simulink model "getTorque"  (R2021a)
settings: Solver=VariableStepAuto  StartTime=0.0  StopTime=10.0  RelTol=1e-3
libraries: cstblocks x1
settings Model: Creator=zande  LastModifiedBy=zande

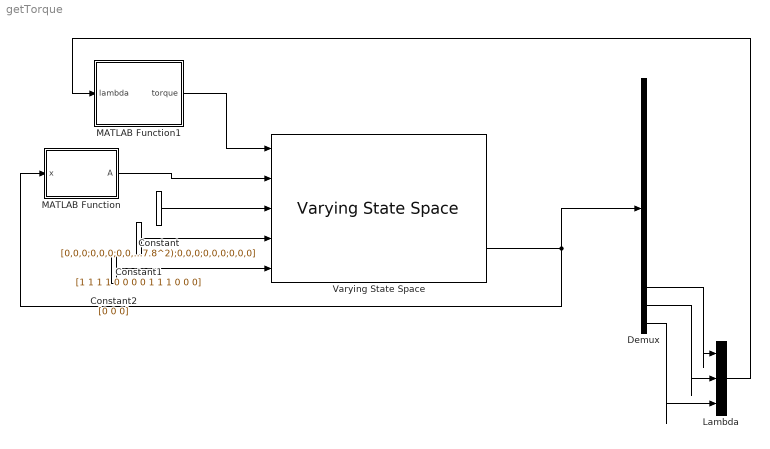
== system getTorque ==
  Constant : Constant  Value=[0,0,0;0,0,0;0,0,0;0,0,0;0,0,0;0,0,0;0,0,0;0,0,0;1/(396.2^2),0,0;0,1/(1867^2),0;0,0,1/(1987.8^2);0,0,0;0,0,0;0,0,0]
  Constant1 : Constant  Value=[1 1 1 1 0 0 0 0 1 1 1 0 0 0]
  Constant2 : Constant  Value=[0 0 0]
  Demux : Demux  Outputs=14
  Lambda : Mux  Inputs=3
  MATLAB Function : MATLAB Function  TreatAsAtomicUnit=on
  MATLAB Function1 : MATLAB Function  TreatAsAtomicUnit=on
  Varying State Space : cstblocks/Linear Parameter Varying/Varying State Space  x0=[2;2;2;2;2;2;.25;.25;.25;.25;.25;.25;2;2]  xNames=''  OutputX=on  OutputDX=off
  wires:
  MATLAB Function/1(A) -> Varying State Space/2
  Varying State Space/2 -> Demux/1, MATLAB Function/1(x)
  Demux/14 -> Lambda/3
  Lambda/1 -> MATLAB Function1/1(lambda)
  MATLAB Function1/1(torque) -> Varying State Space/1
  Constant/1 -> Varying State Space/3
  Constant1/1 -> Varying State Space/4
  Constant2/1 -> Varying State Space/5
  Demux/13 -> Lambda/2
  Demux/12 -> Lambda/1

== matlab function getTorque/MATLAB Function ==
  data: x input size=14;1; A output
function A = A_sim(x)

I1 = 396.2;
I2 = 1867;
I3 = 1987.8;

J1 = (I3 - I2) / I1;
J2 = (I1 - I3)/I2;
J3 = (I2 - I1)/I3;

L1 = -x(12)/I1;
L2 = -x(13)/I2;
L3 = -x(14)/I3;

lambda1 = x(12);
lambda2 = x(13);
lambda3 = x(14);

lambda = [lambda1;lambda2;lambda3];

w1 = x(9);
w2 = x(10);
w3 = x(11);

G = .5 * [0 -w1 -w2 -w3;w1 0 w3 -w2;w2 -w3 0 w1;w3 w2 -w1 0];

B0 = x(1);
B1 = x(2);
B2 = x(3);
B3 = x(4);

Beta = [B0;B1;B2;B3];

Betadot = G * Beta;

Gamma1 = x(5);
Gamma2 = x(6);
Gamma3 = x(7);
Gamma4 = x(8);
gamma = [Gamma1; Gamma2; Gamma3; Gamma4];

w1dot = -J1 * w2 * w3 - lambda1/I1^2;
w2dot = -J2 * w3 * w1 - lambda2/I2^2;
w3dot = -J3 * w1 * w2 - lambda3/I3^2;

omegadot = [w1dot;w2dot;w3dot];

A = [0 -w1/2 -w2/2 -w3/2 0 0 0 0 -B1/2 -B2/2 -B3/2 0 0 0;...
    w1/2 0 w3/2 -w2/2 0 0 0 0 B0/2 -B3/2 B2/2 0 0 0 ;...
    w2/2 -w3/2 0 w1/2 0 0 0 0 B3/2 B0/2 -B1/2 0 0 0;...
    w3/2 w2/2 -w1/2 0 0 0 0 0 -B2/2 B1/2 B0/2 0 0 0;...
    0 0 0 0 0 -w1/2 -w2/2 -w3/2 -Gamma2/2 -Gamma3/2 -Gamma4/2 0 0 0;...
    0 0 0 0 w1/2 0 w3/2 -w2/2 Gamma1/2 -Gamma4/2 Gamma3/2 0 0 0;...
    0 0 0 0 w2/2 -w3/2 0 w1/2 Gamma4/2 Gamma1/2 -Gamma2/2 0 0 0;...
    0 0 0 0 w3/2 w2/2 -w1/2 0  -Gamma3/2 Gamma2/2 Gamma1/2  0 0 0;...
    0 0 0 0 0 0 0 0 0 -603*w3/1981 -604*w2/1981 -7520916276034565/1180591620717411303424 0 0;...
    0 0 0 0 0 0 0 0 (7958*w3)/9335 0 (7958*w1)/9335 0 -2709574194869161/9444732965739290427392 0;...
    0 0 0 0 0 0 0 0 -(7354*w2)/9939 -(7354*w1)/9939 0 0 0 -4780510832214597/18889465931478580854784;...
    -Gamma2/2 Gamma1/2 Gamma4/2 -Gamma3/2 B1/2 -B0/2 -B3/2 B2/2 0 (7354*lambda3)/9939 -(7958*lambda2)/9335 0 -(7958*w3)/9335 (7354*w2)/9939;...
    -Gamma3/2 -Gamma4/2 Gamma1/2 Gamma2/2 B2/2  B3/2 -B0/2 -B1/2  (7354*lambda3)/9939  0   (604*lambda1)/1981 (604*w3)/1981 0 (7354*w1)/9939;...
    -Gamma4/2 Gamma3/2 -Gamma2/2 Gamma1/2 B3/2 -B2/2 B1/2 -B0/2 -(7958*lambda2)/9335 (604*lambda1)/1981 0 (604*w2)/1981 -(7958*w1)/9335 0];

== matlab function getTorque/MATLAB Function1 ==
  data: lambda input size=3;1; torque output
function torque = getTorque(lambda)


I1 = 396.2;
I2 = 1867;
I3 = 1987.8;

L1 = -lambda(1) / I1;
L2 = -lambda(2) / I2;
L3 = -lambda(3) / I3;

torque = [L1;L2;L3];
